simulink model "zadanie_2"  (Simulink 7.7)
settings: Solver=ode4  StartTime=0.0  StopTime=50.0  FixedStep=0.01  RelTol=1e-3
undefined symbols (not defined in the file or in its folder): dfilt, fdesignblkfcn, gcbh
libraries: dsparch4 x2
settings Model: Creator=Aleksander  LastModifiedBy=Jacek
settings DataIOCC: LimitDataPoints=off  SignalLoggingSaveFormat=Dataset
settings OptimizationCC: ExpressionDepthLimit=128
settings CodeAppCC: CustomSymbolStrType=$N$R$M_T
settings GRTTargetCC: CombineOutputUpdateFcns=on

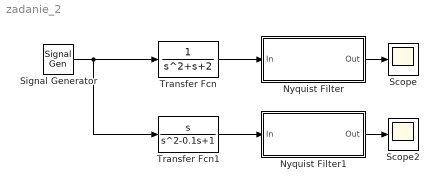
== system zadanie_2 ==
  Nyquist Filter : Subsystem  DialogController=fdesignblkfcn  DialogControllerArgs=DataTag1  InitFcn=fdesignblkfcn(gcbh, {'InitFcn'});
      settings: CopyFcn=fdesignblkfcn(gcbh, {'CopyFcn'});
      mask Type: Nyquist Filter
      mask Description: Design a Nyquist filter
      mask Help: helpview(mapfilelocation('dsp'), 'dspnyquistfilter');
      mask Display: disp('Nyquist');
  Nyquist Filter1 : Subsystem  DialogController=fdesignblkfcn  DialogControllerArgs=DataTag4  InitFcn=fdesignblkfcn(gcbh, {'InitFcn'});
      settings: CopyFcn=fdesignblkfcn(gcbh, {'CopyFcn'});
      mask Type: Nyquist Filter
      mask Description: Design a Nyquist filter
      mask Help: helpview(mapfilelocation('dsp'), 'dspnyquistfilter');
      mask Display: disp('Nyquist');
  Scope : Scope
      settings: TimeRange=50  YMin=-1.5  YMax=1.5
  Scope2 : Scope
      settings: TimeRange=50  YMin=-1.5  YMax=1.5  SaveName=ScopeData2
  Signal Generator : SignalGenerator
  Transfer Fcn : TransferFcn  Denominator=[1 1 2]
  Transfer Fcn1 : TransferFcn  Numerator=[1 0]  Denominator=[1 -0.1 1]
  wires:
  Signal Generator/1 -> Transfer Fcn1/1, Transfer Fcn/1
  Transfer Fcn1/1 -> Nyquist Filter1/1(In)
  Nyquist Filter1/1(Out) -> Scope2/1
  Transfer Fcn/1 -> Nyquist Filter/1(In)
  Nyquist Filter/1(Out) -> Scope/1

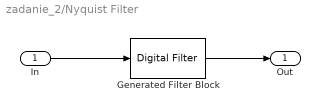
== system zadanie_2/Nyquist Filter ==
  In : Inport
  Generated Filter Block : dsparch4/Digital Filter  Tag=BlockMethodSubSystem  TypePopup=FIR (all zeros)  IIRFiltStruct=Direct form II transposed  AllPoleFiltStruct=Direct form  FIRFiltStruct=Direct form  CoeffSource=Specify via dialog  NumCoeffs=[-1.51622726129956e-05 0 4.1706564279713e-05 0 -8.63974532359493e-05 0 0.000156112339412393 0 -0.000259152163405613 0 0.000405340967727107 0 -0.000606122081126901 0 0.000874664613518895 0 -0.00122600321576426 0 0.00167724728876562 0 -0.0022479153417376 0 0.0029604801760878 0 -0.00384125870473808 0 0.004921861111316 0 -0.0062415564318662 0 0.00785117446710229 0 -0.00981967458384361 0 0.0122455627766693 0 -0.0152776505052993 0 0.0191551639220553 0 -0.0242917549435244 0 0.0314715991488982 0 -0.0423816072426853 0 0.0614206608292716 0 -0.104744991792953 0 0.317854846111936 0.5 0.317854846111936 0 -0.104744991792953 0 0.0614206608292716 0 -0.0423816072426853 0 0.0314715991488982 0 -0.0242917549435244 0 0.0191551639220553 0 -0.0152776505052993 0 0.0122455627766693 0 -0.00981967458384361 0 0.00785117446710229 0 -0.0062415564318662 0 0.004921861111316 0 -0.00384125870473808 0 0.0029604801760878 0 -0.0022479153417376 0 0.00167724728876562 0 -0.00122600321576426 0 0.000874664613518895 0 -0.000606122081126901 0 0.000405340967727107 0 -0.000259152163405613 0 0.000156112339412393 0 -8.63974532359493e-05 0 4.1706564279713e-05 0 -1.51622726129956e-05]  DenCoeffs=[1 0.1]  BiQuadCoeffs=[1 0.3 0.4 1 0.1 0.2]  LatticeCoeffs=[0.2 0.4]  denIgnore=on  FiltPerSampPopup=One filter per frame  IC=0  ICnum=0  ICden=0  roundingMode=Floor  overflowMode=off  ScaleValues=1  scaleValueFracLength=14  stageInFracLength=15  stageOutFracLength=15  FilterSource=Specify via dialog  dfiltObjectName=dfilt.dffir([1 2 1])  InputProcessing=Columns as channels (frame based)
  Out : Outport
  wires:
  In/1 -> Generated Filter Block/1
  Generated Filter Block/1 -> Out/1

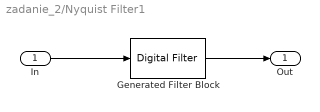
== system zadanie_2/Nyquist Filter1 ==
  In : Inport
  Generated Filter Block : dsparch4/Digital Filter  Tag=BlockMethodSubSystem  TypePopup=FIR (all zeros)  IIRFiltStruct=Direct form II transposed  AllPoleFiltStruct=Direct form  FIRFiltStruct=Direct form  CoeffSource=Specify via dialog  NumCoeffs=[-1.51622726129956e-05 0 4.1706564279713e-05 0 -8.63974532359493e-05 0 0.000156112339412393 0 -0.000259152163405613 0 0.000405340967727107 0 -0.000606122081126901 0 0.000874664613518895 0 -0.00122600321576426 0 0.00167724728876562 0 -0.0022479153417376 0 0.0029604801760878 0 -0.00384125870473808 0 0.004921861111316 0 -0.0062415564318662 0 0.00785117446710229 0 -0.00981967458384361 0 0.0122455627766693 0 -0.0152776505052993 0 0.0191551639220553 0 -0.0242917549435244 0 0.0314715991488982 0 -0.0423816072426853 0 0.0614206608292716 0 -0.104744991792953 0 0.317854846111936 0.5 0.317854846111936 0 -0.104744991792953 0 0.0614206608292716 0 -0.0423816072426853 0 0.0314715991488982 0 -0.0242917549435244 0 0.0191551639220553 0 -0.0152776505052993 0 0.0122455627766693 0 -0.00981967458384361 0 0.00785117446710229 0 -0.0062415564318662 0 0.004921861111316 0 -0.00384125870473808 0 0.0029604801760878 0 -0.0022479153417376 0 0.00167724728876562 0 -0.00122600321576426 0 0.000874664613518895 0 -0.000606122081126901 0 0.000405340967727107 0 -0.000259152163405613 0 0.000156112339412393 0 -8.63974532359493e-05 0 4.1706564279713e-05 0 -1.51622726129956e-05]  DenCoeffs=[1 0.1]  BiQuadCoeffs=[1 0.3 0.4 1 0.1 0.2]  LatticeCoeffs=[0.2 0.4]  denIgnore=on  FiltPerSampPopup=One filter per frame  IC=0  ICnum=0  ICden=0  roundingMode=Floor  overflowMode=off  ScaleValues=1  scaleValueFracLength=14  stageInFracLength=15  stageOutFracLength=15  FilterSource=Specify via dialog  dfiltObjectName=dfilt.dffir([1 2 1])  InputProcessing=Columns as channels (frame based)
  Out : Outport
  wires:
  In/1 -> Generated Filter Block/1
  Generated Filter Block/1 -> Out/1
